simulink model "VEHICLE_DYN_TRAIN"  (R2019b)
settings: Solver=ode4  StartTime=0.0  StopTime=150  FixedStep=0.01  RelTol=1e-3
model workspace (MAT data in the model file):
  ACCEL = [0 0.000975932898663 -0.0414538855996 0.0440661905922 -0.0484817487001 0.0392964510644 -0.0693895143615 0.0261566921783 -0.0586295561215 0.0249771458914 -0.0595081132089 0.0233316013131 ... (544 elements, 17x32)]
  A_mc = 0.000491
  CMD_BR = [0 0 0 0 0 0 0 0 0 0 0 0 ... (15001 elements, 15001x1)]
  CMD_MODE = [1 1 1 1 1 1 1 1 1 1 1 1 ... (15001 elements, 15001x1)]
  CMD_ST = [0 0 0 0 0 0 0 0 0 0 0 0 ... (15001 elements, 15001x1)]
  CMD_T = [0 0.01 0.02 0.03 0.04 0.05 0.06 0.07 0.08 0.09 0.1 0.11 ... (2001 elements, 1x2001)]
  CMD_TH = [0 0 0 0 0 0 0 0 0 0 0 0 ... (15001 elements, 15001x1)]
  CMD_TM = [0 0.01 0.02 0.03 0.04 0.05 0.06 0.07 0.08 0.09 0.1 0.11 ... (15001 elements, 15001x1)]
  CMD_U = [10 10 10 10 10 10 10 10 10 10 10 10 ... (2001 elements, 1x2001)]
  CMD_UX = [0.1 0.1 0.1 0.1 0.1 0.1 0.1 0.1 0.1 0.1 0.1 0.1 ... (15001 elements, 15001x1)]
  COMMAND = [0 0 0 0 0 0 0 0 0 0 0 0 ... (102 elements, 17x6)]
  C_q = 1.4e-06
  DATA_HMMWV : object (value not decoded)
  DATA_VESIM_CC_BRAKE : object (value not decoded)
  FORCE = [0 -4628.45620853 2357.84853747 -1841.82564621 -1727.75397473 1695.19792057 -1263.06335256 1524.31841051 -1649.98396845 -1537.1025145 -1335.96213703 1639.88309903 ... (493 elements, 17x29)]
  F_cf = 80
  F_cs = 138
  F_z = -50097.6
  Gain_v = 70
  J_wheel = 32
  K_vb = 1500
  Kp_rpm = 2.7013
  Kp_v = 30
  L3 = 10
  MIN_TH = 0
  M_sprung = 4672
  M_unsprung = 220
  M_unsprung_front = 220
  M_vehicle = 5112
  N2 = 0
  N3 = 0.01
  P = 36
  P_0 = 10670
  P_gain = 0.0006
  R_wheel = 0.4412
  SLIP = [0 -0.5 0.5 -0.5 -0.5 0.5 -0.5 0.5 -0.5 -0.5 -0.5 0.5 ... (136 elements, 17x8)]
  STATE = [0 4.33747954961e-06 -0.000147430460781 -3.72129119222e-05 -0.000284189368187 -0.000207128204422 -0.00055150808757 -0.000594561033148 -0.000967775941564 -0.00103412952076 -0.00143215770154 -0.00152470872631 ... (544 elements, 17x32)]
  STATES_INIT = [0 0 0.9902452 0 0 1.57079632679 0.01 0 0 0 0 0 ... (32 elements, 1x32)]
  SUSP = [0 -0.00875795294893 -0.00878173856984 -0.00830852863719 -0.00873591176348 -0.00870428588158 -0.00751721170558 -0.00851904716693 -0.00789923296531 -0.00838039895253 -0.00756270047902 -0.00866403364289 ... (612 elements, 17x36)]
  S_o = 3
  T2_r = 4
  TIRE = [0 0.0910654620457 -0.0936729683319 0.0717372732987 0.0513932148365 -0.0365035701266 -0.00739813929507 -0.0045484168787 0.0723881675257 0.0296400174207 -0.0169805208571 0.0207214713062 ... (408 elements, 17x24)]
  TIRELIFTOFF = [0 0 0 0 0 0 0 0 0 0 0 0 ... (17 elements, 17x1)]
  T_LENGTH = 2001
  T_STEP = 0.01
  T_STOP = 12.82
  T_TOTAL = 20
  Ti_rpm = 0.6464
  Ti_v = 2.5
  Tstop = [150 150 150 150 150 150 150 150 150 150 150 150 ... (15001 elements, 15001x1)]
  Tt_rpm = 0.0808
  Tt_v = 0.3125
  U_INIT = 0.01
  b = 170
  brake_Pw = [-3.96235801772 -3.96238075942 -0.895107722214 -0.895547395081 35.9159438465 72.7273668629 152.485661058 244.514654481 330.408495385 364.152342142 462.316700341 535.939857177 ... (40 elements, 40x1)]
  brake_V = [-1.14468402636e-08 6.09303685082e-09 2.9257815427e-07 6.31682445149e-07 8.18779962309e-07 1.05849711081e-06 1.41515318379e-06 1.67826507702e-06 1.8361367918e-06 2.02323385108e-06 2.22788040303e-06 2.46760304614e-06 ... (40 elements, 40x1)]
  diff_efficiency = 0.94
  diff_wRatio = 6.052
  diff_w_ratio = 3.56
  end_time = 140
  engine_inertia = 0.53
  fmin_mg = [42.75 43.31 51.6 64.3 73.65 71.1 72.7 72.36]
  fmin_mg_na = [42.79 42.79 42.79 42.79 42.79 42.79 42.79 42.79]
  g = -9.8
  g_motor_eff = 1
  gr_motor = 0
  i = 5
  mdot_fuel = [5e-06 1e-05 2e-05 3e-05 4e-05 5e-05 6e-05 7e-05 8e-05]
  ms2mph = 2.23694
  n_tire = 4
  no_cyl = 8
  num_points = 14000
  num_points_fast = 140000
  rpm0 = 83.7758040957
  rpm0_c = 1000
  rpm2rads = 0.10471975512
  rpm_e = [50 800 1000 1500 2000 2500 3000 3300]
  rpm_engine = [700 800 1000 1500 2000 2500 3000 3300]
  rpm_hi_idle = 3400
  rpm_idle = 750
  rpm_max_c = 3200
  rpm_rated = 3200
  start_time = 0
  time_step = 0.01
  time_step_fast = 0.001
  torque_engine = [9.767 15.303 12.411 -4.524 -12.214 -35.77 -70 -75.889 75.383 80.318 76.501 61.314 ... (72 elements, 8x9)]
  tout = [0 0.01 0.02 0.03 0.04 0.05 0.06 0.07 0.08 0.09 0.1 0.11 ... (17 elements, 17x1)]
  trq_scale = 0.46
values from neighbouring files (symbols this model uses):
  B = Ref(i:i+2,2)    [Calc_vref.m]    (also in Parameter_load.m = 0.1; VEHICLE_DYN_TRAIN_INIT.m = 0.25)
  Error_now = Error_now_array(end)    [RUN_SIMULATION_SHARED_NEW_POWERTRAIN.m]    (also in VEHICLE_DYN_TRAIN_INIT.m = 0)
  J = 0.075    [VEHICLE_DYN_TRAIN_INIT.m]
  K = 0.075    [VEHICLE_DYN_TRAIN_INIT.m]
  pid2tau_gain = 2.5    [VEHICLE_DYN_TRAIN_INIT.m]
  st_a_in = st_sc_out(end)    [RUN_SIMULATION_SHARED_NEW_POWERTRAIN.m]    (also in VEHICLE_DYN_TRAIN_INIT.m = 0)
  tau_a_in = tau_a_out(end)    [RUN_SIMULATION_SHARED_NEW_POWERTRAIN.m]    (also in VEHICLE_DYN_TRAIN_INIT.m = 0)
undefined symbols (not defined in the file or in its folder): adaptive_flag, autonomy_human_contain_gain, Bias_Distance, dt, error_lookuptable, human_autonomy_agreement_threshold, human_contain_min, human_response_dead_zone, human_torque_max, J_cal, kp_sc, model_lookuptable, Standard_Devices, steering_stable_threshold, UDP_Protocol, vdes, Xobs, Yobs
libraries: simulink x16, sldrtlib x3, dspstat3 x3, vrlib x2
(part 4 of 4)

== matlab function VEHICLE_DYN_TRAIN/Haptic Shared Control/Subsystem2/MATLAB Function ==
  data: theta input; thetad input; athetadd input; F_p output
function F_p = force_prediction(theta, thetad, athetadd)
% bi-section
init_1 = -0.4228;
init_2 = 0.4386;
sol_tol = 0.0001;

while abs(init_1 - init_2) > sol_tol
    med = (init_1 + init_2)/2;
    if abs(generate_solution(init_1, theta, athetadd, thetad)) < 0.0001
        init_2 = init_1;
    elseif abs(generate_solution(init_2, theta, athetadd, thetad)) < 0.0001
        init_1 = init_2;
    elseif generate_solution(init_1, theta, athetadd, thetad)*generate_solution(med, theta, athetadd, thetad) <= 0
        init_2 = med;
    else
        init_1 = med;
    end
end
F_p = (init_1 + init_2)/2;

    function sol = generate_solution(F, theta, athetadd, thetad)
        sol = F + athetadd - generate_b(F, theta)*thetad;
    end

    function b = generate_b(F, theta)
        eval_F = [-0.70 ,-0.60, -0.57, -0.55, -0.52, -0.50, -0.47, -0.45, -0.42, -0.40, -0.39, -0.38, -0.37, -0.36, -0.35, -0.34, -0.33, -0.32, -0.31, -0.30, -0.29, -0.28, -0.27, -0.26, -0.25, -0.24, -0.23, -0.22, -0.21, -0.20, -0.19, 0.17, 0.18, 0.19, 0.20, 0.21, 0.22, 0.23, 0.24, 0.25, 0.26, 0.27, 0.28, 0.29, 0.30, 0.31, 0.32, 0.33, 0.34, 0.35, 0.36, 0.37, 0.38, 0.39, 0.40, 0.42, 0.45, 0.47, 0.50, 0.52, 0.55, 0.57, 0.60];
        eval_F = eval_F + ((eval_F<0).*+0.1772 + (eval_F>0).*-0.1614);
        eval_theta = [-0.16, -0.15, -0.13, -0.11, -0.09, -0.07, -0.05, -0.03, -0.01, 0, 0.01, 0.03, 0.05, 0.07, 0.09, 0.11, 0.13, 0.15, 0.16];
        b_ref = [...
            7.0467, 5.2850, 3.5233, 2.7277, 2.4252, 2.2078, 1.9896, 2.1133, 1.4272, 1.4464, 1.8675, 1.6168, 1.9454, 2.1594, 2.3480, 2.7159, 3.5293, 4.9741, 10.5700;...%-0.70
            7.0467, 5.2850, 3.5233, 2.7277, 2.4252, 2.2078, 1.9896, 2.1133, 1.4272, 1.4464, 1.8675, 1.6168, 1.9454, 2.1594, 2.3480, 2.7159, 3.5293, 4.9741, 10.5700;...%-0.60
            6.0431, 4.9100, 3.2733, 2.8057, 2.1523, 2.1348, 1.7575, 1.7497, 1.6411, 1.6134, 1.6238, 1.7115, 1.8705, 1.9838, 2.3312, 2.6187, 3.0659, 5.2373, 10.2933;...%-0.57
            6.2133, 5.3257, 3.2256, 2.5710, 2.2250, 2.0372, 1.8230, 1.6423, 1.5415, 1.5213, 1.5313, 1.6387, 1.7966, 1.7923, 2.2323, 2.5710, 3.1954, 4.9707, 7.4560;...%-0.55
            6.8560, 3.9111, 2.9809, 2.3641, 2.1235, 1.9151, 1.5653, 1.5653, 1.5325, 1.4172, 1.4612, 1.5582, 1.6887, 1.7055, 2.0239, 2.4486, 3.1164, 4.5707, 8.5700;...%-0.52
            6.4560, 4.3040, 2.9345, 2.3057, 2.0430, 1.8446, 1.6554, 1.5102, 1.3914, 1.3884, 1.4220, 1.4541, 1.6221, 1.7834, 2.0826, 2.3911, 2.8070, 4.4524, 7.4492;...%-0.50
            4.8800, 3.9927, 2.6618, 2.0914, 1.9013, 1.5853, 1.5411, 1.4283, 1.3225, 1.3035, 1.2944, 1.3910, 1.5250, 1.6358, 1.9520, 2.0914, 2.4618, 4.1829, 7.7600;...%-0.47
            6.8200, 3.4100, 2.6231, 2.0985, 1.6934, 1.6884, 1.4826, 1.3438, 1.2595, 1.2495, 1.2485, 1.3147, 1.4588, 1.5333, 1.8187, 2.0224, 2.7280, 3.7628, 6.8200;...%-0.45
            4.8560, 3.4686, 2.3124, 1.8677, 1.6687, 1.3679, 1.3640, 1.2451, 1.1444, 1.1283, 1.1453, 1.1961, 1.3196, 1.4715, 1.6716, 1.8677, 2.4280, 3.4686, 5.3956;...%-0.42
            4.4560, 3.1829, 2.2280, 1.7138, 1.5690, 1.3288, 1.2731, 1.1726, 1.0226, 1.0665, 1.0900, 1.1367, 1.2117, 1.4101, 1.5201, 1.8567, 2.2280, 3.7133, 4.0509;...%-0.40
            4.5106, 3.5467, 2.1280, 1.6369, 1.4986, 1.3641, 1.2160, 1.1141, 0.9372, 1.0109, 0.9776, 1.0885, 1.1955, 1.2251, 1.4812, 1.7733, 2.1280, 3.0400, 5.3200;...%-0.39
            4.3800, 3.3800, 1.9314, 1.8436, 1.5364, 1.4182, 1.2675, 1.1523, 1.0562, 1.0496, 1.0607, 1.1122, 1.2291, 1.3703, 1.5600, 1.6900, 2.0280, 3.3800, 6.7600;...%-0.38
            9.6400, 3.2133, 1.9280, 1.7527, 1.5424, 1.3251, 1.2280, 1.1209, 1.0377, 1.0145, 1.0205, 1.0955, 1.1803, 1.2205, 1.5224, 1.7527, 2.1100, 3.0560, 6.8200;...%-0.37
            9.1400, 3.0467, 2.2850, 1.6618, 1.4862, 1.3642, 1.2106, 1.1012, 1.0184, 0.9779, 1.0270, 1.0381, 1.1794, 1.2151, 1.4822, 1.6618, 2.2850, 3.0060, 5.5700;...%-0.36
            4.3200, 3.4560, 2.1600, 1.7280, 1.5429, 1.4400, 1.2706, 1.1597, 1.0654, 1.0378, 1.0673, 1.0148, 1.2432, 1.3606, 1.6000, 1.7280, 2.1600, 3.2560, 5.7600;...%-0.35
            8.1400, 3.2560, 2.0350, 1.6280, 1.5654, 1.4157, 1.2921, 1.1587, 1.0682, 1.0365, 1.0696, 1.0926, 1.2241, 1.3681, 1.5505, 1.6089, 2.3257, 3.2560, 5.4267;...%-0.34
            5.0933, 3.0560, 2.1829, 1.6978, 1.5434, 1.4018, 1.2628, 1.1319, 1.0596, 1.0349, 1.0480, 1.0685, 1.2031, 1.3287, 1.5280, 1.6978, 2.1829, 3.0560, 5.0933;...%-0.33
            4.7600, 2.8560, 2.0400, 1.7850, 1.4875, 1.2865, 1.2102, 1.0901, 1.0340, 0.9882, 1.0099, 1.0200, 1.1802, 1.3346, 1.4875, 1.7850, 2.0400, 3.1733, 4.7600;...%-0.32
            5.3120, 2.9511, 2.4560, 1.7707, 1.5810, 1.4593, 1.3020, 1.2893, 0.9124, 1.0703, 1.2051, 1.1021, 1.1964, 1.3621, 1.7826, 1.8971, 2.0145, 3.0271, 6.6400;...%-0.31
            6.1400, 2.7289, 2.2327, 1.7543, 1.7175, 1.2792, 1.2926, 1.1423, 1.0285, 1.0422, 1.1825, 1.0586, 1.1922, 1.3569, 1.5336, 1.7543, 2.0467, 3.0086, 4.9120;...%-0.30
            3.7600, 3.0229, 2.2260, 1.7500, 1.5040, 1.3756, 1.2129, 1.2261, 0.9956, 0.9907, 1.0236, 0.9616, 1.1510, 1.2966, 1.3429, 1.7905, 2.0560, 3.0878, 5.6400;...%-0.29
            6.2800, 3.2267, 2.0560, 1.7133, 1.6062, 1.4899, 1.2850, 1.1953, 1.0576, 1.0388, 1.0708, 1.0821, 1.2094, 1.3892, 1.5118, 1.8691, 2.2844, 3.2267, 5.1400;...%-0.28
            4.6400, 3.2400, 2.2622, 1.7467, 1.6000, 1.4730, 1.3449, 1.2052, 1.1127, 1.0941, 1.1317, 1.1317, 1.2541, 1.4061, 1.6000, 1.8560, 2.3200, 3.0933, 4.6400;...%-0.27
            4.1400, 2.7600, 2.0700, 1.7700, 1.5923, 1.4526, 1.2738, 1.1500, 1.1753, 1.0336, 1.1355, 1.0753, 1.2795, 1.2938, 1.5623, 1.7560, 2.1700, 2.8600, 5.1400;...%-0.26
            3.6400, 2.9120, 1.8200, 1.4560, 1.3736, 1.1648, 1.2661, 0.9973, 0.9455, 0.8999, 0.9122, 0.9455, 1.0628, 1.1742, 1.3736, 1.8200, 2.0800, 2.9120, 3.6400;...%-0.25
            3.1400, 3.1400, 2.0933, 1.5700, 1.4273, 1.2816, 1.2077, 1.0555, 0.9508, 0.9191, 0.9458, 0.9662, 1.0467, 1.1849, 1.3802, 1.5700, 2.0933, 2.0933, 6.2800;...%-0.24
            5.2800, 2.6400, 1.7600, 1.3200, 1.3538, 1.2878, 1.2000, 1.0154, 0.9412, 0.9085, 1.0312, 0.9263, 1.0154, 1.1234, 1.2878, 1.7600, 1.7600, 2.6400, 4.6400;...%-0.23
            6.4800, 2.1400, 1.4267, 1.4267, 1.2970, 1.0700, 1.0974, 0.9304, 0.7329, 0.8013, 0.8231, 0.7782, 0.9106, 1.0439, 1.1889, 1.4267, 1.4267, 2.1400, 6.4800;...%-0.22
            4.6800, 2.1867, 1.6400, 1.3120, 1.0933, 1.0092, 1.0933, 0.8000, 0.7736, 0.6961, 0.7472, 0.6979, 0.7904, 0.8865, 1.0754, 1.0933, 1.3120, 2.1867, 4.6800;...%-0.21
            4.5600, 2.2800, 1.3680, 1.1400, 1.0688, 1.0364, 1.0133, 0.7475, 0.7475, 0.6598, 0.7331, 0.6706, 0.7125, 0.8769, 1.0364, 1.1400, 1.1400, 2.2800, 4.5600;...%-0.20
            2.5600, 1.9200, 1.2800, 0.8533, 0.8000, 0.7529, 0.8000, 0.5818, 0.5447, 0.4288, 0.5110, 0.4491, 0.5020, 0.6095, 0.7420, 0.8533, 1.2800, 1.2800, 2.8400;...%-0.19
            
            0.9801, 0.8696, 0.6484, 0.4987, 0.4596, 0.4598, 0.4465, 0.3984, 0.3501, 0.3501, 0.3501, 0.3984, 0.4465, 0.4598, 0.4596, 0.4987, 0.6484, 0.8696, 0.9801;...
            1.9013, 1.6674, 1.1997, 0.8794, 0.7967, 0.8043, 0.7629, 0.6781, 0.5997, 0.5997, 0.5997, 0.6781, 0.7629, 0.8043, 0.7967, 0.8794, 1.1997, 1.6674, 1.9013;...
            2.0337, 1.8431, 1.4617, 1.1568, 1.0182, 0.9695, 0.9481, 0.8350, 0.7578, 0.7578, 0.7578, 0.8350, 0.9481, 0.9695, 1.0182, 1.1568, 1.4617, 1.8431, 2.0337;...
            2.7919, 2.4495, 1.7646, 1.3272, 1.1971, 1.1264, 1.0362, 0.9966, 0.9079, 0.9079, 0.9079, 0.9966, 1.0362, 1.1264, 1.1971, 1.3272, 1.7646, 2.4495, 2.7919;...
            2.6983, 2.4057, 1.8203, 1.3931, 1.2182, 1.1377, 1.0665, 0.9688, 0.8972, 0.8972, 0.8972, 0.9688, 1.0665, 1.1377, 1.2182, 1.3931, 1.8203, 2.4057, 2.6983;...
            2.8268, 2.4864, 1.8054, 1.4162, 1.3061, 1.1838, 1.0953, 0.9767, 0.9612, 0.9612, 0.9612, 0.9767, 1.0953, 1.1838, 1.3061, 1.4162, 1.8054, 2.4864, 2.8268;...
            2.8584, 2.5726, 2.0009, 1.5802, 1.3832, 1.2587, 1.1828, 1.0554, 1.0217, 1.0217, 1.0217, 1.0554, 1.1828, 1.2587, 1.3832, 1.5802, 2.0009, 2.5726, 2.8584;...
            3.1268, 2.7998, 2.1458, 1.6240, 1.3987, 1.3380, 1.2281, 1.1229, 1.1032, 1.1032, 1.1032, 1.1229, 1.2281, 1.3380, 1.3987, 1.6240, 2.1458, 2.7998, 3.1268;...
            3.0939, 2.8127, 2.2502, 1.7899, 1.5427, 1.4063, 1.3126, 1.1836, 1.1684, 1.1684, 1.1684, 1.1836, 1.3126, 1.4063, 1.5427, 1.7899, 2.2502, 2.8127, 3.0939;...
            3.4414, 3.0741, 2.3394, 1.7942, 1.5645, 1.4607, 1.3507, 1.2325, 1.1952, 1.1952, 1.1952, 1.2325, 1.3507, 1.4607, 1.5645, 1.7942, 2.3394, 3.0741, 3.4414;...
            3.2580, 2.9865, 2.4435, 1.8965, 1.5765, 1.4877, 1.3834, 1.2852, 1.2567, 1.2567, 1.2567, 1.2852, 1.3834, 1.4877, 1.5765, 1.8965, 2.4435, 2.9865, 3.2580;...
            2.9194, 2.6457, 2.0983, 1.6849, 1.4794, 1.3477, 1.2419, 1.1404, 1.1459, 1.1459, 1.1459, 1.1404, 1.2419, 1.3477, 1.4794, 1.6849, 2.0983, 2.6457, 2.9194;...
            3.2287, 2.9003, 2.2437, 1.7614, 1.5376, 1.3978, 1.2796, 1.1534, 1.2036, 1.2036, 1.2036, 1.1534, 1.2796, 1.3978, 1.5376, 1.7614, 2.2437, 2.9003, 3.2287;...
            3.3586, 3.0139, 2.3247, 1.8108, 1.5683, 1.4215, 1.3075, 1.2158, 1.2260, 1.2260, 1.2260, 1.2158, 1.3075, 1.4215, 1.5683, 1.8108, 2.3247, 3.0139, 3.3586;...
            2.9721, 2.7244, 2.2290, 1.7890, 1.5295, 1.3953, 1.2866, 1.2383, 1.2425, 1.2425, 1.2425, 1.2383, 1.2866, 1.3953, 1.5295, 1.7890, 2.2290, 2.7244, 2.9721;...
            3.4207, 3.0320, 2.2546, 1.7260, 1.4961, 1.3162, 1.2439, 1.1662, 1.2200, 1.2200, 1.2200, 1.1662, 1.2439, 1.3162, 1.4961, 1.7260, 2.2546, 3.0320, 3.4207;...
            3.2041, 2.8989, 2.2887, 1.7759, 1.5120, 1.3992, 1.2677, 1.1832, 1.2836, 1.2836, 1.2836, 1.1832, 1.2677, 1.3992, 1.5120, 1.7759, 2.2887, 2.8989, 3.2041;...
            3.2228, 2.8871, 2.2157, 1.7518, 1.5386, 1.3686, 1.2446, 1.1711, 1.2725, 1.2725, 1.2725, 1.1711, 1.2446, 1.3686, 1.5386, 1.7518, 2.2157, 2.8871, 3.2228;...
            3.0441, 2.7794, 2.2500, 1.8127, 1.5556, 1.3868, 1.2700, 1.1899, 1.2573, 1.2573, 1.2573, 1.1899, 1.2700, 1.3868, 1.5556, 1.8127, 2.2500, 2.7794, 3.0441;...
            3.0736, 2.7780, 2.1869, 1.7530, 1.5345, 1.3744, 1.2731, 1.1648, 1.1540, 1.1540, 1.1540, 1.1648, 1.2731, 1.3744, 1.5345, 1.7530, 2.1869, 2.7780, 3.0736;...
            3.0118, 2.7329, 2.1753, 1.7180, 1.4749, 1.3458, 1.2199, 1.1557, 1.2307, 1.2307, 1.2307, 1.1557, 1.2199, 1.3458, 1.4749, 1.7180, 2.1753, 2.7329, 3.0118;...
            3.1563, 2.8641, 2.2795, 1.8063, 1.5536, 1.4103, 1.2821, 1.2035, 1.3169, 1.3169, 1.3169, 1.2035, 1.2821, 1.4103, 1.5536, 1.8063, 2.2795, 2.8641, 3.1563;...
            3.4738, 3.0816, 2.2972, 1.8250, 1.6502, 1.4607, 1.3939, 1.2630, 1.3607, 1.3607, 1.3607, 1.2630, 1.3939, 1.4607, 1.6502, 1.8250, 2.2972, 3.0816, 3.4738;...
            3.4012, 3.0696, 2.4064, 1.8896, 1.6348, 1.4959, 1.3557, 1.3074, 1.4815, 1.4815, 1.4815, 1.3074, 1.3557, 1.4959, 1.6348, 1.8896, 2.4064, 3.0696, 3.4012;...
            3.3487, 3.0668, 2.5030, 2.0545, 1.7957, 1.6112, 1.4693, 1.3792, 1.5550, 1.5550, 1.5550, 1.3792, 1.4693, 1.6112, 1.7957, 2.0545, 2.5030, 3.0668, 3.3487;...
            4.0084, 3.6076, 2.8058, 2.2011, 1.8973, 1.6976, 1.5901, 1.4724, 1.6255, 1.6255, 1.6255, 1.4724, 1.5901, 1.6976, 1.8973, 2.2011, 2.8058, 3.6076, 4.0084;...
            4.1272, 3.7126, 2.8834, 2.2985, 2.0152, 1.7890, 1.5948, 1.5240, 1.6681, 1.6681, 1.6681, 1.5240, 1.5948, 1.7890, 2.0152, 2.2985, 2.8834, 3.7126, 4.1272;...
            4.5238, 4.0440, 3.0844, 2.4310, 2.1407, 1.9076, 1.6846, 1.6397, 1.7968, 1.7968, 1.7968, 1.6397, 1.6846, 1.9076, 2.1407, 2.4310, 3.0844, 4.0440, 4.5238;...
            4.7290, 4.2519, 3.2976, 2.5859, 2.2411, 2.0203, 1.8677, 1.7366, 1.8974, 1.8974, 1.8974, 1.7366, 1.8677, 2.0203, 2.2411, 2.5859, 3.2976, 4.2519, 4.7290;...
            5.3025, 4.6965, 3.4845, 2.6168, 2.2838, 2.1410, 2.0187, 1.8287, 1.9626, 1.9626, 1.9626, 1.8287, 2.0187, 2.1410, 2.2838, 2.6168, 3.4845, 4.6965, 5.3025;...
            5.2534, 4.6697, 3.5023, 2.6938, 2.3666, 2.1619, 1.9228, 1.8658, 1.9739, 1.9739, 1.9739, 1.8658, 1.9228, 2.1619, 2.3666, 2.6938, 3.5023, 4.6697, 5.2534;...
            5.6391, 5.0126, 3.7595, 2.8304, 2.4448, 2.2784, 2.1395, 1.9668, 2.0836, 2.0836, 2.0836, 1.9668, 2.1395, 2.2784, 2.4448, 2.8304, 3.7595, 5.0126, 5.6391;
            ];
        %         idx = min(find(F<=eval_F));
        %         jdx = min(find(theta<=eval_theta));
        if F < -0.60
            F = -0.60;
        end
        if F > 0.60
            F = 0.60;
        end
        if theta < -0.158
            theta = -0.158;
        end
        if theta > 0.158
            theta = 0.158;
        end
        
        Fx = find(F<=eval_F);
        
        if isempty(Fx)
            
            idx = length(eval_F);
            
        else
            
            idx = min(Fx);
            
        end
        
        Ft = find(theta<=eval_theta);
        
        if isempty(Ft)
            
            jdx = length(eval_theta);
            
        else
            
            jdx = min(Ft);
        end
        if F == eval_F(idx)
            b_ref_u = b_ref(idx, :);
        else
            b_ref_u = b_ref(idx-1,:) + (b_ref(idx,:)-b_ref(idx-1,:))/(eval_F(idx)-eval_F(idx-1))*(F-eval_F(idx-1));
        end
        if theta == eval_theta(jdx)
            b = b_ref_u(jdx);
        else
            b = b_ref_u(jdx-1) + (b_ref_u(jdx)-b_ref_u(jdx-1))/(eval_theta(jdx)-eval_theta(jdx-1))*(theta-eval_theta(jdx-1));
        end
    end

end

== matlab function VEHICLE_DYN_TRAIN/Vehicle System/Subsystem/MATLAB Function2 ==
  data: X0 input; ST_length input; X0predicted output; SP_length input; time_step input; idx input; dt input; st_old input; sp_old input
function X0predicted = fcn(X0, ST_length, SP_length, time_step, idx, dt, st_old, sp_old)
x0 = X0(1);
y0 = X0(2);
vy0 = X0(3);
dpsi = X0(4);
psi = X0(5);
if time_step == 0
    X0predicted = X0;
else
    if idx >= 1 
        st = ST_length(idx);
        vdes = SP_length(idx);
    else
        st = st_old;
        vdes = sp_old;
    end
    for i = 1:time_step
        four_dot = dotcalculator(st,vdes,x0,y0,vy0,dpsi,psi);
        if idx + i > 101
            st = ST_length(101);
            vdes = SP_length(101);
        else
            st = ST_length(idx+i);
            vdes = SP_length(idx+i);
        end
        x0 = x0 + dt * four_dot(1);
        y0 = y0 + dt * four_dot(2);
        vy0 = vy0 + dt * four_dot(3);
        dpsi = dpsi + dt * four_dot(4);
        psi = psi + dt * dpsi;
    end
    if idx + time_step > 101
        X0predicted = [x0; y0; vy0; dpsi; psi; ST_length(101); SP_length(101); 0];
    else
        a = idx+time_step;
        if a > 1
            X0predicted = [x0; y0; vy0; dpsi; psi; ST_length(a); SP_length(a); (SP_length(a) - SP_length(a-1))/dt];
        elseif a == 1
            X0predicted = [x0; y0; vy0; dpsi; psi; ST_length(a); SP_length(a); (SP_length(a) - sp_old)/dt];
        else
            X0predicted = [x0; y0; vy0; dpsi; psi; st_old; sp_old; (sp_old - vdes)/dt];
        end
    end
end
  


function fourdot = dotcalculator(st,vdes,x0,y0,vy0,dpsi,psi)
    % define model parameters
    m          = 2.6887e+03;
    Izz        = 4.1101e+03;
    la         = 1.5775;      % distance from CoG to front axle
    lb         = 1.7245;        % distance from CoG to rear axle
    FzF0       = 1.3680e+04;
    FzR0       = 1.2696e+04;
    dFzx_coeff = 705.;
    KZX        = 705.;
    KZYR       = 1040.;

    % defines polynominal for acceleration bounds
    AXC= [-0.000128015180401862,	0.00858618595422724,	-0.225657108071454,	3.08283259993589,	-0.000138537090018958,	0.00684702729623608,	-0.120391102052425,	-3.55886697370079];

    % vehicle Limits
    x_min    = 0.;
    x_max    = 400.;
    y_min    = 0.;
    y_max    = 400.;
    sa_min   = -30*pi/180;
    sa_max   = 30*pi/180;
    psi_min  = -2*pi;
    psi_max  = 2*pi;
    u_min    = 5.;   %5.
    u_max    = 29.;
    sr_min   = -5*pi/180;
    sr_max   = 5*pi/180;
    jx_min   = -5.;
    jx_max   = 5.;

    % tire parameters
    FZ0     = 35000.0;
    PCY1    = 1.5874;               %Shape factor Cfy for lateral forces
    PDY1    = 0.73957;              %Lateral friction Muy
    PDY2    = -0.075004;            %Variation of friction Muy with load
    PEY1    = 0.37562;              %Lateral curvature Efy at Fznom
    PEY2    = -0.069325;            %Variation of curvature Efy with load
    PEY3    = 0.29168;              %Zero order camber dependency of curvature Efy
    PKY1    = -10.289;              %Maximum value of stiffness Kfy/Fznom
    PKY2    = 3.3343;               %Load at which Kfy reaches maximum value
    PHY1    = 0.0056509;            %Horizontal shift Shy at Fznom
    PHY2    = -0.0020257;           %Variation of shift Shy with load
    PVY1    = 0.015216;             %Vertical shift in Svy/Fz at Fznom
    PVY2    = -0.010365;            %Variation of shift Svy/Fz with load
    PC1     = PCY1;
    PD1     = PDY1 - PDY2;
    PD2     = PDY2/FZ0;
    PE1     = PEY1 - PEY2;
    PE2     = PEY2/FZ0;
    PE3     = PEY3;
    PK1     = PKY1*FZ0;
    PK2     = 1/(PKY2*FZ0);
    PH1     = PHY1 - PHY2;
    PH2     = PHY2/FZ0;
    PV1     = PVY1 - PVY2;
    PV2     = PVY2/FZ0;

    Caf =  -8.4138e+04;	% cornering stiffness--front axle (N/rad)
    Car =  -7.8126e+04;	% cornering stiffness-- rear axle (N/rad)
    Fyf_min = -7500;
    Fyf_max = 7500;
    % constrained initial states
    x0_     = 0.;
    y0_     = 0.;
    psi0_   = 0.8464;
    v0_     = 0.;
    u0_     = 10.;
    sa0_    = 0.;
    sr0_    = 0.;
    ax0_    = 0.;
    jx0_    = 0.;
    r0_     = 0.;

    %%TODO: Move some of these parameters somewhere else
    % weights
    w_goal = 1.; % should be zero when vehicle is not within goal distance during prediction horizon
    w_psi  = 0.01;
    w_time = 0.05;
    w_haf  = 1.0e-5;
    w_Fz   = 0.1;  %0.5 in paper
    w_ce   = 1.;
    w_sa   = 0.1;
    w_sr   = 1.;
    w_jx   = 0.01;

    sm      = 5.; % (m) distance to make sure we don't hit obstacle
    Fz_min  = 1000.;
    Fz_off  = 100.;
    a_t     = Fz_min + 3*Fz_off;  % soft tire force constraint constants
    b_t     = Fz_off;
    EP      = 0.001;

    % other parameters
    L_Rd      = 5.;       % relaxation constant for LiDAR range (m)
    L_R       = 100.;     % LiDAR range (m)
    sigma     = 1.;       % 0.05 (m)small margin, if the vehicle is within this margin, then the target is considered to be reached

    
r=dpsi;    
v=vy0;    
ax=0;
ux=vdes;
sa=st;
FYF=( (PD2*(FzF0 - (ax - v*r)*dFzx_coeff)^2 + PD1*(FzF0 - (ax - v*r)*dFzx_coeff))*sin(PC1*atan((((PK1*sin(2*atan(PK2*(FzF0 - (ax - v*r)*dFzx_coeff))))/(((PD2*PC1*(FzF0 - (ax - v*r)*dFzx_coeff)^2 + PD1*PC1*(FzF0 - (ax - v*r)*dFzx_coeff)) + ((PD2*PC1*(FzF0 - (ax - v*r)*dFzx_coeff)^2 + PD1*PC1*(FzF0 - (ax - v*r)*dFzx_coeff)))/(((PD2*PC1*(FzF0 - (ax - v*r)*dFzx_coeff)^2 + PD1*PC1*(FzF0 - (ax - v*r)*dFzx_coeff))^2 + EP^2)^(0.5))*0.001)+EP))*((atan((v + la*r)/(ux+EP)) - sa) + PH2*(FzF0 - (ax - v*r)*dFzx_coeff) + PH1)) - ((PE2*(FzF0 - (ax - v*r)*dFzx_coeff) + PE1)*(1 - PE3)*(((atan((v + la*r)/(ux+EP)) - sa) + PH2*(FzF0 - (ax - v*r)*dFzx_coeff) + PH1))/((((atan((v + la*r)/(ux+EP)) - sa) + PH2*(FzF0 - (ax - v*r)*dFzx_coeff) + PH1)^2 + EP^2)^(0.5)))*((((PK1*sin(2*atan(PK2*(FzF0 - (ax - v*r)*dFzx_coeff))))/(((PD2*PC1*(FzF0 - (ax - v*r)*dFzx_coeff)^2 + PD1*PC1*(FzF0 - (ax - v*r)*dFzx_coeff)) + ((PD2*PC1*(FzF0 - (ax - v*r)*dFzx_coeff)^2 + PD1*PC1*(FzF0 - (ax - v*r)*dFzx_coeff)))/(((PD2*PC1*(FzF0 - (ax - v*r)*dFzx_coeff)^2 + PD1*PC1*(FzF0 - (ax - v*r)*dFzx_coeff))^2 + EP^2)^(0.5))*0.001)+EP))*((atan((v + la*r)/(ux+EP)) - sa) + PH2*(FzF0 - (ax - v*r)*dFzx_coeff) + PH1)) - atan((((PK1*sin(2*atan(PK2*(FzF0 - (ax - v*r)*dFzx_coeff))))/(((PD2*PC1*(FzF0 - (ax - v*r)*dFzx_coeff)^2 + PD1*PC1*(FzF0 - (ax - v*r)*dFzx_coeff)) + ((PD2*PC1*(FzF0 - (ax - v*r)*dFzx_coeff)^2 + PD1*PC1*(FzF0 - (ax - v*r)*dFzx_coeff)))/(((PD2*PC1*(FzF0 - (ax - v*r)*dFzx_coeff)^2 + PD1*PC1*(FzF0 - (ax - v*r)*dFzx_coeff))^2 + EP^2)^(0.5))*0.001)+EP))*((atan((v + la*r)/(ux+EP)) - sa) + PH2*(FzF0 - (ax - v*r)*dFzx_coeff) + PH1)))))) + (PV2*(FzF0 - (ax - v*r)*dFzx_coeff)^2 + PV1*(FzF0 - (ax - v*r)*dFzx_coeff)));
FYR=( (PD2*(FzR0 + (ax - v*r)*dFzx_coeff)^2 + PD1*(FzR0 + (ax - v*r)*dFzx_coeff))*sin(PC1*atan((((PK1*sin(2*atan(PK2*(FzR0 + (ax - v*r)*dFzx_coeff))))/(((PD2*PC1*(FzR0 + (ax - v*r)*dFzx_coeff)^2 + PD1*PC1*(FzR0 + (ax - v*r)*dFzx_coeff)) + ((PD2*PC1*(FzR0 + (ax - v*r)*dFzx_coeff)^2 + PD1*PC1*(FzR0 + (ax - v*r)*dFzx_coeff)))/(((PD2*PC1*(FzR0 + (ax - v*r)*dFzx_coeff)^2 + PD1*PC1*(FzR0 + (ax - v*r)*dFzx_coeff))^2+EP^2)^(0.5))*0.001)+EP))*((atan((v - lb*r)/(ux+EP))) + PH2*(FzR0 + (ax - v*r)*dFzx_coeff) + PH1)) - ((PE2*(FzR0 + (ax - v*r)*dFzx_coeff) + PE1)*(1 - PE3*(((atan((v - lb*r)/(ux+EP))) + PH2*(FzR0 + (ax - v*r)*dFzx_coeff) + PH1))/((((atan((v - lb*r)/(ux+EP))) + PH2*(FzR0 + (ax - v*r)*dFzx_coeff) + PH1)^2 + EP^2)^(0.5))))*((((PK1*sin(2*atan(PK2*(FzR0 + (ax - v*r)*dFzx_coeff))))/(((PD2*PC1*(FzR0 + (ax - v*r)*dFzx_coeff)^2 + PD1*PC1*(FzR0 + (ax - v*r)*dFzx_coeff)) + ((PD2*PC1*(FzR0 + (ax - v*r)*dFzx_coeff)^2 + PD1*PC1*(FzR0 + (ax - v*r)*dFzx_coeff)))/(((PD2*PC1*(FzR0 + (ax - v*r)*dFzx_coeff)^2 + PD1*PC1*(FzR0 + (ax - v*r)*dFzx_coeff))^2+EP^2)^(0.5))*0.001)+EP))*((atan((v - lb*r)/(ux+EP))) + PH2*(FzR0 + (ax - v*r)*dFzx_coeff) + PH1)) - atan((((PK1*sin(2*atan(PK2*(FzR0 + (ax - v*r)*dFzx_coeff))))/(((PD2*PC1*(FzR0 + (ax - v*r)*dFzx_coeff)^2 + PD1*PC1*(FzR0 + (ax - v*r)*dFzx_coeff)) + ((PD2*PC1*(FzR0 + (ax - v*r)*dFzx_coeff)^2 + PD1*PC1*(FzR0 + (ax - v*r)*dFzx_coeff)))/(((PD2*PC1*(FzR0 + (ax - v*r)*dFzx_coeff)^2 + PD1*PC1*(FzR0 + (ax - v*r)*dFzx_coeff))^2+EP^2)^(0.5))*0.001)+EP))*((atan((v - lb*r)/(ux+EP))) + PH2*(FzR0 + (ax - v*r)*dFzx_coeff) + PH1)))))) + (PV2*(FzR0 + (ax - v*r)*dFzx_coeff)^2 + PV1*(FzR0 + (ax - v*r)*dFzx_coeff)));
FZ_rl_con=(  0.5*(FzR0 + KZX*(ax - v*r)) - KZYR*((FYF + FYR)/m) - Fz_min);
FZ_rr_con=( 0.5*(FzR0 + KZX*(ax - v*r)) + KZYR*((FYF + FYR)/m) - Fz_min);



  xdot = ( vdes*cos(psi) - (v + la*r)*sin(psi));      % X position
  ydot= ( vdes*sin(psi) + (v + la*r)*cos(psi));        % Y position
  vydot = ((FYF + FYR)/m - r*ux);                    % Lateral Speed
  psiddot= ((la*FYF-lb*FYR)/Izz);                           % Yaw Rate
  fourdot=[xdot,ydot,vydot,psiddot];
end
end

== matlab function VEHICLE_DYN_TRAIN/Haptic Shared Control/Subsystem2/MATLAB Function1 ==
  data: F input; b input; J_cal input; theta_p output; theta input; thetad input; dt input
function theta_p = theta_prediction(F, b, J_cal, theta, thetad, dt)
    if b == 0 
        b = 10;
    end
    c_2 = (thetad-(F/b))/(-b/J_cal);
    c_1 = theta - c_2;
    theta_p = c_1 + c_2 * exp((-b/J_cal)*dt) + F/b*dt;
end

== matlab function VEHICLE_DYN_TRAIN/Haptic Shared Control/torque conversion/MATLAB Function ==
  data: x1 input; yout output
function yout  = fitNet_v5_br(x1)
%FITNET_V5_BR neural network simulation function.
%
% Auto-generated by MATLAB, 01-Apr-2020 15:18:04.
%
% [y1] = fitNet_v5_br(x1) takes these arguments:
%   x = 1xQ matrix, input #1
% and returns:
%   y = 1xQ matrix, output #1
% where Q is the number of samples.

%#ok<*RPMT0>

autonomy_torque_thres=0.125;

if abs(x1(end))<=autonomy_torque_thres
    yout=0;
else
    % ===== NEURAL NETWORK CONSTANTS =====
    x1=x1';
    
    % Input 1
    x1_step1.xoffset = -0.59;
    x1_step1.gain = 1.69491525423729;
    x1_step1.ymin = -1;
    
    % Layer 1
    b1 = [0.3123601105165873526;-0.30317543057648471683;3.8014021554231294253;0.31811219769250037581;-0.30634401998767119002;0.30541984286955803363;-0.30684786468496566547;-0.29593680327258514717;-0.29812768132245021091;0.29679639962289722233;-0.29560576494307849726;0.29479828081839443144;-0.2925116458249872875;-0.32600042435329779078;-0.29074798432105131152;0.28662686924048935699;0.28461623571509586661;0.28173489872817647495;-0.28304182106754854908;-0.28112355364558200277;0.27641101040847587678;-0.35198488783254450185;0.047511421725580066378;0.2751049607937821051;0.27274989541367083978;-0.27978194349357971005;-0.27802550644584772543;-0.29003254515570375816;0.28947611140531770424;0.4093437433649310675;0.099378831294478053859;0.42483872481664441967;0.37144942949288456413;0.18205092543332668242;-0.41752911655992558382;-0.10451517944215585332;-0.1524573289006266319;0.54628196799950501372;-0.55440574353806293395;-0.83745375850925973804;0.76393144460003270524;-0.67201420946408008117;-0.61953421929248952971;-0.51565373639399791905;-0.22142558435538051143;0.68932125835973323547;0.60345829603962475307;-0.21520246053519656582;-0.15508608691463332541;0.35992603032830794429;-0.21876189306017754244;0.32018037942458621448;-0.16522557212334496035;0.083641772723770935194;-0.66918465911310520688;-0.29454085603984114794;-1.2752309610120213801;0.17132323028905349638;0.19311164915575163015;-0.281406351030930868;-0.23884378326512431534;0.21204065946249012198;0.21280951048504115342;-0.21477317119611505358;-0.22227565395576426299;0.23125964551075420261;-0.2350168005253427117;-0.23033988604096389263;-0.22465266426991131743;0.20964390871703439401;0.18260536227733692449;0.15337296028769256684;-0.13162683182722734188;0.073487369273545113946;-0.11204317026579128924;0.023455024511174218937;0.045871993195491705952;-0.14056431446601933;-0.17900255976648921097;-0.048148057480962090648;0.047833772825568797449;0.034871783313103948965;0.020688443049998724715;-0.016764575538395658227;-0.012521042180544212849;-0.0094539166588114738332;-0.0066920855411911487134;-0.007653678561785303737;-0.0031793660948182802736;-0.0021715091985117333795;-0.0037492632903832036687;0.0056730161395377688358;0.011023175006176321247;-0.012974055198726811011;-0.014510251261313717244;-0.022096849579157810256;-0.022508082042193153921;-0.020803775345208837255;-0.22957675726345883049;0.0031251290129651358371;-0.023497008202247166714;-0.19358022358141785402;-0.6243306546921799649;0.31416925240508630779;-0.10643076979555227135;0.0020373446065838807413;-0.33695398393909414825;-0.20805480779511068001;0.10408394242192883783;-0.004589386905566454275;0.050671002149626345745;0.85758751319523562895;0.14481933809395067247;0.077317623702850224454;0.30379060842477001447;-0.51535013459696066285;0.2092030666393748517;-0.16847479822860658705;2.2528395767489581836;-0.57952630400352966866;-0.17476658314996790233;-0.089721142687638241742;0.77719497940764992183;-0.10835280257356860734;0.13573542627785975534;0.071530117078330207603;-0.028711678540026066425;-0.20520489675760542059;-0.033535114644390892624;-0.42938129990359324983;0.14545928287678652757;-0.4881764518306168088;0.22278688273573010736;-0.59655850022297762791;0.42591827827612954716;0.18381840967097792805;0.17837987068730465356;-0.088485417182156259064;0.16051554972184858827;-0.1069614607035552778;-0.18245765710176886643;0.1654784506513675979;0.79010670879679656409;0.21210607543231593808;0.21106196853028472149;-0.21416115024945020506;-0.21149309431491006284;-0.45315933891068244099;-0.20051051032604388924;0.22215647397191562451;-0.2166554112556807743;0.51007799563290812106;-0.25661765768834576829;0.26102151110170640491;-0.30574533406037573968;-0.26053669185796979324;-0.58023120816552420376;-0.52779406972831754974;-0.56949312387209705122;0.66473082785395742889;-0.66853434951705148492;-0.67668336692356045869;0.56034625715984154315;-0.65968892165124737303;0.89223620864968988808;1.0111875879624410146;0.61416884295778195746;-0.47690170786718821816;1.0320400819699466766;-0.13620749288771596963;0.36223383929305030815;-1.3308852672299431585;-1.209786056555027578;1.4582763404545093788;-1.3111954952783455575];
    IW1_1 = [-0.57099637047702633819;0.66719867471864757746;6.784906666833916411;-0.8020902719039209039;0.6826333947516736167;-0.62716984045665236103;0.59702516045797449085;0.58865342816409305104;0.55325229132904807372;-0.55146498949308475623;0.55218031171026882298;-0.54874869428236527913;0.54280983221911549563;0.41682320739467149107;0.54598230271719916384;-0.50317051351669439541;-0.50303021318210738855;-0.51098178583447528833;0.50334626077600230776;0.50176998286404550509;-0.50812701187611053477;0.49591239017533439437;-0.67025824242128706487;-0.50861936222013959252;-0.51936190943135496223;0.59419632496711594083;0.48171566881914257285;0.58941832043966624344;-0.49309766895528361896;-0.09435334006334057666;-0.69710548294072149922;-0.5657296227581445347;0.82822547241863575529;-0.55546584596250170307;-0.83690685178764678831;0.49086399866359431421;-0.55228539100100548787;0.95651498150616687255;-0.022248112311569527566;-0.20459091322085609654;0.14941631367725297097;-0.069494131337827252937;-0.018955420286511592831;0.097423615643060679226;0.1389118034723683115;1.0728406405483079666;0.015214979528948301829;0.46933088783196846849;0.76630740179814071933;-0.80980555455634151141;0.87505458073993158674;-0.81881286981018075455;0.78548891697037115378;-0.73946248797785263385;-0.10771521952625388863;-0.19042343228123065346;2.899622026545380038;0.024783355582378801402;0.14982456853369480188;-0.12616910641042697327;0.44443693533822192787;-0.45404923880185671381;-0.45204071145982410718;0.44890317783738992174;0.44962863162478883261;-0.45920367262361660998;0.47800554956314017518;0.49019484388898210137;0.50083343561606730177;-0.51105941087706030501;-0.52715644212894796627;-0.54388028699800416987;0.54344511658698135825;-0.54556165689964286614;0.53852892917384542759;-0.56237704957064704736;-0.55437656071216745435;0.54503371398966360406;0.46264685715384801235;0.53254834646911031193;-0.53682136546547332134;-0.53902460298335275191;-0.54768149535564503161;0.54795350679157883711;0.54561419241959008275;0.54409477293209995707;0.54190521689752313428;0.54435148327923954525;0.54121008066594389341;-0.53678564409529083701;-0.53667686957704874295;0.53545641080035510928;0.5317561751998091113;-0.53123479639689119569;-0.5304008707384409993;-0.525850597212463855;-0.52624916282280476132;-0.52938143762750189403;0.49617184518113022218;-0.5495460739849832299;-0.52279259330336602662;0.32517228929536606818;-0.24067474083103557181;-0.76513578288342598555;-0.45091443692098853724;-0.55673879427453853985;-0.35049913341855226667;0.82885048103813208087;-0.66160766120506819821;0.5635316931021611131;0.51250319513652897729;0.74139959337070515666;0.65560140636655073187;0.29768621007836720826;0.58600971644127697324;-0.29283808521959425741;0.54019030528183775708;-0.74707190639790110875;0.19499137703072616512;-0.093704209901866730714;-0.48331806030029778043;-0.49460274550788596581;-0.1891439104703292462;-0.46541163838077687087;0.48031091570338363406;0.57281764180043104329;0.62318822163045484164;-0.53084597768394936601;-0.52040637256602062521;-0.46367153404733568722;0.48250885157583750518;-0.2011719185130629306;-0.45075503049866544325;-0.073421786364284008508;0.46167361503160847525;0.48886593094127306358;0.47214494091167658052;-0.58085618177232323234;0.47422308634108689684;-0.51991369366302009336;-0.47331743231434375563;0.36434637069866104842;-1.9960621720919291544;0.47169782248013147896;0.46881017954075576704;-0.48093656068602780307;-0.47716576658847803527;-0.18678795642492473927;-0.52346568153929196043;0.4874516865484053163;-0.47738286727975931534;0.13549930718838487653;-0.45701482173191165792;0.45140369917760542195;-0.41982858012088780653;-0.47956573670717045355;-0.050479040271765050762;-0.12598579464352641089;-0.059773989000081108325;-0.098271846144625918384;0.13302742651705865007;0.14249096428427296401;0.4432020381926767838;-2.4483397208530672806;-1.691564920749315748;-2.214582006201800457;-1.6298618576331174168;1.3623395535962603553;-0.79355764511225101998;0.89234029032467399034;0.36165437305307368554;0.81735167099876804286;0.69960158474152600583;-0.93700541948754501043;0.7485688995050543415];
    
    % Layer 2
    b2 = [0.58093968587967448336;0.38526047084779446728];
    LW2_1 = [-0.002224755018804032685 0.059425699055682873473 -4.8633831866288330659 -0.12357376046382510804 0.063954151004167333894 -0.035968476389585481157 0.019748807208425166182 0.028179971226016682639 0.009572495371269312478 -0.010218660822349212233 0.011741284294800476834 -0.010920300510357869653 0.010496063073189286149 -0.071592146365993758472 0.013690689367913439975 0.00075071594320023048164 -0.0011483430484304532442 -0.007504953572412250383 0.002739578448632498664 0.0039807365845708521379 -0.011344054026919580397 -0.070202448853913496096 -0.39474542137890633597 -0.012742318992137064218 -0.019839602136771813945 0.047786026304135163778 -0.0020749928659020843054 0.033888312229569748923 0.0083011903348194828606 0.24557719804544206332 -0.36436157180403683231 0.13043220463068375126 0.37612121315204694039 -0.12630764455576640182 -0.37132788772376673636 0.15736582192495698895 -0.34398930267817517947 0.30408819357083827217 -0.38532787406421292742 -0.54564451837185146132 0.5163855096610533435 -0.46258343379867089551 -0.42257155830316139866 -0.32402488228749604104 -0.10914165427645985962 0.21222764016292283706 0.41311198752168476478 0.049995004449756380582 0.36027639834777613892 -0.063015891747785504617 0.36667315492237517738 -0.13147918412954520684 0.36240986761958327023 -0.42586856810281403796 -0.46489507870345525564 -0.30864104963101857138 -0.2076641032623436911 0.097440902123480346853 0.227089848858542942 -0.26845884565773098229 0.0093683915144473391134 -0.042110109661982739193 -0.03999811599935067935 0.037758118669349749474 0.033546462640015810297 -0.03335609469629306767 0.043943066338588528119 0.063702953390143160495 0.080269797116409025151 -0.10711686216769912561 -0.1502508553985500428 -0.19467855680079440561 0.21944558747056147618 -0.28186261509145060788 0.23841957434400132265 -0.3476617363184744125 -0.31673877059871913264 0.21103008571407505523 0.085544962585133957345 0.29173192289690791368 -0.29612230122922961195 -0.31224999926806812356 -0.3362611681558159149 0.34078171097249781996 0.34320727190557281938 0.34496126118961062401 0.34588895358887128406 0.34677091498862627761 0.34868632484403566663 -0.35029021172203528289 -0.35164697447683324061 0.35246722888316689426 0.35458343310666606829 -0.35591801702452080525 -0.35671011567367744144 -0.36011558493423012628 -0.3607976731949579241 -0.36157691474673470111 0.044807022743488689187 -0.35459965174401009147 -0.35841640946587333127 0.017005453761198496831 -0.51812083879200099279 -0.10846935823168718516 -0.37662649779893647706 -0.36101543152666015768 -0.46231227516522466203 0.34512226072705110003 -0.33823410830166944496 0.3637482591786405095 0.37477624535094217206 0.80364414043376164454 0.62998939344410409547 0.23074039550816446975 0.70944072726856022282 -0.53789957380016917288 0.56407429624904126264 -0.7575218018565349487 0.72059887379303988464 -0.37637140283875941682 -0.46163610405802701919 -0.3896323084254538216 0.43768028559311578096 -0.38061298075338401148 0.4192287362915590454 0.45565403512811181175 0.38709692013567686963 -0.49059238470961274992 -0.35345584760847409411 -0.66567362257923157198 0.42589092362238978318 -0.48094139492536724934 0.0047381230153501078042 -0.48031058496509493327 0.65657726911649449963 0.46694169221747866549 0.44943866764637896427 -0.47455479414748963363 0.42754108660857004232 -0.42600931045876394565 -0.4485761538943014437 0.31619170111485073171 -0.18684205335153727945 0.4734390432185696107 0.46842652225791303611 -0.48426792966774223625 -0.47748589822997650201 -0.40988419548165400119 -0.51908858946401115197 0.49757971523475591491 -0.47945007489996221972 0.42228990361824342292 -0.49303266703467779619 0.48998355761490003379 -0.4960723477279213034 -0.52076025841730722021 -0.42638877906718986033 -0.42633888188823321208 -0.41630209260916639646 0.40747138182164061027 -0.40447282640176424051 -0.40730578139603262899 0.62348795789095956543 -1.93628785214223198 0.26954117781972852796 0.24453652723247321088 -0.49369438353156014365 0.53779423471344622865 0.27064815067803638104 0.46679782349353238224 0.48406431225394752627 -0.53146057526349166356 -0.51561595140711835583 0.54473311991407524779 -0.53570050502522692515;0.60345490698584958178 -0.68625275628084725366 0.17446332440241182904 0.82252279580792597713 -0.70583380865232980828 0.65719285047088915608 -0.63031804546392511401 -0.61101856749690075521 -0.57933745391410917946 0.57734323816514210304 -0.57796819446617919702 0.57467429570899053459 -0.56717660262272351357 -0.46537001942464190085 -0.57171198684174340254 0.52532376838321759305 0.52491539833307621077 0.53083730065667167342 -0.52456783372351001304 -0.52272439360436229183 0.5263510771101611585 -0.5788020269828471065 0.51538175660614160556 0.52839355567601820063 0.53809093560153553604 -0.61710484305221446899 -0.50512185356993488661 -0.62268015459140835244 0.52618917937606324298 0.14057574417339122053 0.58950871045757313738 0.75202142984305098139 -0.012316528777233971825 0.52631807417007059335 -0.06419341381158853721 -0.40507551589579865459 0.20413017970533375856 0.12708281058206888359 -0.098920270557756387331 -0.17020530685018381289 0.2114478936279189647 -0.2320577886589264005 -0.24492291360639537046 -0.28658791144408429785 -0.2131134130230331325 0.2065499890722207188 0.23820071633138006906 -0.47951313528640221451 -0.71427472009084880256 0.96736116399270988264 -0.8468306323266011626 0.81192819711109609493 -0.73381055652210247509 0.67737886774354705288 0.14386165937597272801 0.20999818058623545558 -3.5591158549166777014 -0.071950329088833711588 -0.14348734899871407045 0.10957721579129449385 -0.46432422468417117178 0.4603959026606436189 0.45926417414604281397 -0.45691389767968193514 -0.46054552353283001453 0.4723062090277910241 -0.4891334762261629332 -0.49370750487436648735 -0.49921222353819871831 0.49952793463397104912 0.49942483111396018813 0.49995507930704474742 -0.48827945701932479183 0.45855050222631615897 -0.47302997489513437523 0.44288649024149501221 0.45016710112672758681 -0.49438850111366000606 -0.45251008523218549939 -0.43504309099153037899 0.43862833996640265832 0.43239568420450485986 0.43043963038137411647 -0.42832140328723422584 -0.4236459849421020385 -0.42070172840545205784 -0.41704664618090708794 -0.42067111237985782557 -0.41496471545042390439 0.40750013521057854016 0.40689595079648538389 -0.40467577187778325243 -0.39797945700035208816 0.39674063499513417819 0.39490643683593312785 0.38636425075641556148 0.38659457003370073513 0.39164714414976170564 -0.50773315543080288492 0.42603333659998088301 0.38108363101238001969 -0.30191514773616873191 -0.2443431662895648171 0.8232718347077684351 0.24479793682264100463 0.43690059072004228113 -0.036956233983501292351 -0.82336060572147728998 0.6067539248122468809 -0.44596796679088945847 -0.35059054571680225987 0.1550441145855222802 -0.37932908324715103321 -0.1995447757111315501 -0.19178653271726500695 -0.14509019641296563852 -0.25703629863528870692 0.40861427400529271026 0.34723401650303592492 -0.23145939994714403998 0.25031002637729121707 0.31808155106230201481 0.10419629872532201742 0.28736318190574300369 -0.27654039761505366801 -0.38446632167872535346 -0.48717294789976522962 0.23616990109283458876 0.37188929137790893709 -0.036753346082960644536 -0.2695694987786474428 -0.12227201733697390384 0.45978716941388886319 -0.390782601063635604 0.033901791351105374506 -0.2444740094077399728 -0.24073369237633354678 0.37338129744360332163 -0.25277434164544365647 0.31934120769175544652 0.23677724605754976728 -0.18587659977248219279 1.9858495711725672184 -0.21357322261675740216 -0.21229780843769102683 0.216805701506768006 0.21639056530606531892 -0.10152643058688717859 0.25065487521601148568 -0.2139487055501023971 0.21196019770025653628 0.16819165689518464357 0.16965849100204546951 -0.16290948597858356806 0.11028024390290459833 0.17783858954616521553 -0.25087167580392161215 -0.17579920343897800783 -0.24032948200419618212 0.36071362890097680154 -0.49148889822100394476 -0.53769981952823464599 0.32313037189665760884 -0.26155546788960726268 0.9205474452847113298 1.7384199280721728265 1.7783024295349800781 -1.5436137313843161234 0.16883033876396999484 -0.719828057497053031 -0.13217792627142654904 -0.30512941253090958282 -0.32999878003677124427 0.29241011577376330166 -0.75425087584640848615];
    
    % Layer 3
    b3 = 0.39374064516651141599;
    LW3_2 = [0.017913588998011192172 -0.014293701205371090596];
    
    % Output 1
    y1_step1.ymin = -1;
    y1_step1.gain = 0.0755561946922233;
    y1_step1.xoffset = -18.578629013;
    
    % ===== SIMULATION ========
    
    % Dimensions
    Q = size(x1,2); % samples
    
    % Input 1
    xp1 = bsxfun(@minus,x1,x1_step1.xoffset);
    xp1 = bsxfun(@times,xp1,x1_step1.gain);
    xp1 = bsxfun(@plus,xp1,x1_step1.ymin);
    
    % Layer 1
    a1 = 2 ./ (1 + exp(-2*(repmat(b1,1,Q) + IW1_1*xp1))) - 1;
    
    % Layer 2
    a2 = 2 ./ (1 + exp(-2*(repmat(b2,1,Q) + LW2_1*a1))) - 1;
    
    % Layer 3
    % a3 = 2 ./ (1 + exp(-2*(repmat(b3,1,Q) + LW3_2*a2))) - 1;
    a3 = repmat(b3,1,Q) + LW3_2*a2;
    
    % % Layer4
    % a4 = repmat(b4,1,Q) + LW4_3*a3;
    
    % Output 1
    y1 = bsxfun(@minus,a3,y1_step1.ymin);
    % y1 = bsxfun(@minus,a4,y1_step1.ymin);
    y1 = bsxfun(@rdivide,y1,y1_step1.gain);
    y1 = bsxfun(@plus,y1,y1_step1.xoffset);
    
    thres=10;
    if abs(y1(length(y1)))<thres
        yout=y1(length(y1));
    else
        yout=sign(y1(length(y1)))*thres;
    end
end

end

== matlab function VEHICLE_DYN_TRAIN/Haptic Shared Control/Force Generator/Adaptive block/MATLAB Function ==
  data: T input; y output; sigma input
function y = new_shared_control_scheme(T, sigma)

%% phase 1 setting parameter
    node1 = 5;
    node2 = 45;
    max_ass = 1;
    min_ass = 0.1;
    min_thre = 0.01;
    max_thre = 0.3;
    alpha = 0.1;
    
    f = (max_ass-min_ass) * exp(12/abs(node2-node1)*(abs(sigma-50)-abs(50-(node1+node2)/2)))./(exp(12/abs(node2-node1)*(abs(sigma-50)-abs(50-(node1+node2)/2)))+1)+min_ass;
    g = (max_thre-min_thre)/2500*(sigma-50).^2+min_thre;
    h = 0.6-g;
    y = 1-(1-f)*exp(12/h*(abs(T)-g-h/2))./(exp(12/h*(abs(T)-g-h/2))+1);
end

== matlab function VEHICLE_DYN_TRAIN/Haptic Shared Control/human ST 2 Tau/MATLAB Function ==
  data: tau_a_in input; tau_h output; st_h input; kp_sc input; dead_zone input; k_c input; threshold input; human_contain input; omega_st input; theta_st input; Error_now input
function tau_h  = humanSteering2Torque(tau_a_in, st_h, kp_sc, dead_zone, k_c, threshold, human_contain, omega_st, theta_st, Error_now)

tau_h=0;
tau_h_contain=k_c*sign(tau_a_in)*(abs(tau_a_in)-dead_zone);
tau_h_modify=kp_sc*(st_h-theta_st);

sign_h=sign(st_h-theta_st);
sign_a=sign(tau_a_in);

if sign_h~=sign_a && abs(st_h-theta_st) > threshold
    if abs(st_h-theta_st) > threshold
        tau_h=-tau_a_in+tau_h_modify;
    elseif omega_st>human_contain % Steering wheel rotates too fast
        tau_h=tau_h_contain;
    else
        tau_h=0;
    end
end

end
